simulink model "aufg2_schaltbild2"  (R2015a)
settings: Solver=ode45  StartTime=0.0  StopTime=10.0  RelTol=1e-3
settings Model: Creator=Daniel  LastModifiedBy=Daniel

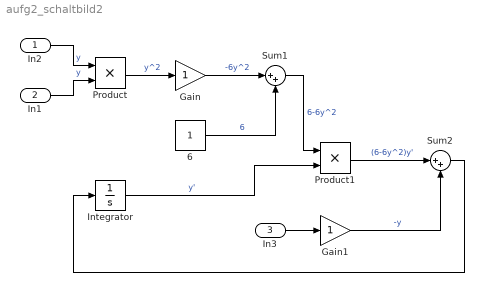
== system aufg2_schaltbild2 ==
  In2 : Inport
  In1 : Inport  Port=2
  In3 : Inport  Port=3
  6 : Constant
  Gain : Gain
  Gain1 : Gain
  Integrator : Integrator
  Product : Product
  Product1 : Product
  Sum1 : Sum  Inputs=|++
  Sum2 : Sum  Inputs=|++
  wires:
  Integrator/1 -> Product1/2  "y'"
  In2/1 -> Product/1  "y"
  In1/1 -> Product/2  "y"
  Product/1 -> Gain/1  "y^2"
  Gain/1 -> Sum1/1  "-6y^2"
  6/1 -> Sum1/2  "6"
  Sum1/1 -> Product1/1  "6-6y^2"
  In3/1 -> Gain1/1
  Product1/1 -> Sum2/1  "(6-6y^2)y'"
  Gain1/1 -> Sum2/2  "-y"
  Sum2/1 -> Integrator/1
